simulink model "io_vector_size"  (Simulink 10.1)
settings: Solver=FixedStepDiscrete  StartTime=0.0  StopTime=10.0  RelTol=1e-3  EnableMultiTasking=on
settings Model: Creator=Demo  LastModifiedBy=MaximeBe
settings DataIOCC: LimitDataPoints=on  SaveFormat=Dataset
settings OptimizationCC: ZeroExternalMemoryAtStartup=off  ZeroInternalMemoryAtStartup=off  LifeSpan=auto
settings DebuggingCC: UnderspecifiedInitializationDetection=Simplified  MergeDetectMultiDrivingBlocksExec=error  AllowSymbolicDim=off  SFExecutionAtInitializationDiag=warning
settings HardwareCC: ProdBitPerPointer=64  ProdBitPerSizeT=64  ProdBitPerPtrDiffT=64  ProdLargestAtomicFloat=Float  ProdIntDivRoundTo=Zero  ProdEndianess=LittleEndian  ProdWordSize=64  ProdHWDeviceType=Intel->x86-64 (Windows64)
settings RTWCC: Description=Generate an RTMaps component embedding the model  SystemTargetFile=rtmaps.tlc  TemplateMakefile=rtmaps_default_tmf  PostCodeGenCommand=rtmaps_post_code_generation(buildInfo)  RetainRTWFile=on  TargetLang=C++
settings STFCustomTargetCC: ModelReferenceCompliant=off  ConcurrentExecutionCompliant=on  CombineOutputUpdateFcns=on  MultiInstanceERTCode=on  CodeInterfacePackaging=C++ class  CPPClassGenCompliant=on  GRTInterface=off  SystemTargetFile=rtmaps.tlc
settings GRTTargetCC: ModelReferenceCompliant=off  ParMdlRefBuildCompliant=off  CompOptLevelCompliant=off  CombineOutputUpdateFcns=on  MatFileLogging=off  MultiInstanceERTCode=on  CodeInterfacePackaging=C++ class  GRTInterface=off  UseToolchainInfoCompliant=off
settings CPPComponent: GenerateDestructor=on  ExternalIOMemberVisibility=private  GenerateExternalIOAccessMethods=Inlined structure-based method  ParameterMemberVisibility=public  InternalMemberVisibility=private  GenerateParameterAccessMethods=None  GenerateInternalMemberAccessMethods=None  UseOperatorNewForModelRefRegistration=off  IncludeModelTypesInModelClass=on

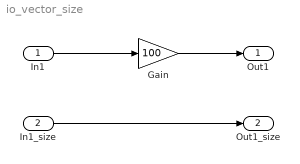
== system io_vector_size ==
  In1 : Inport  OutDataTypeStr=double  PortDimensions=10
  In1_size : Inport  Port=2  OutDataTypeStr=int32  PortDimensions=1
  Gain : Gain  Gain=100
  Out1 : Outport  OutDataTypeStr=double  PortDimensions=10
  Out1_size : Outport  Port=2  OutDataTypeStr=int32  PortDimensions=1
  wires:
  In1/1 -> Gain/1
  Gain/1 -> Out1/1
  In1_size/1 -> Out1_size/1
